simulink model "Simulink_Assem"  (R2023a)
settings: Solver=VariableStepAuto  StartTime=0.0  StopTime=10.0  RelTol=1e-3
libraries: dspsigops x1
settings Model: Creator=assem  LastModifiedBy=assem

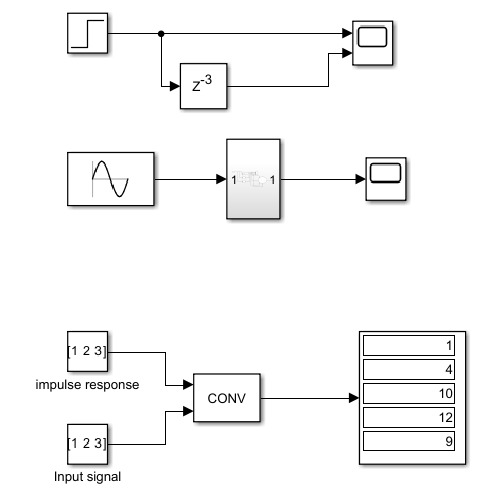
[thumbnail: Simulink's stored preview of the top-level diagram]
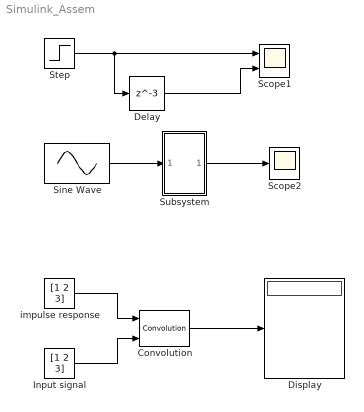
== system Simulink_Assem ==
  Convolution : dspsigops/Convolution  domain=Time  roundingMode=Floor  overflowMode=off  outputDataTypeStr=Inherit: Same as accumulator  outputMin=[]  outputMax=[]  outputLastDataTypeStr=Inherit: Same as accumulator
  Delay : Delay  DelayLength=3
  Display : Display
  Input signal : Constant  Value=[1 2 3]
  Scope1 : Scope  NumInputPorts=2
  Scope2 : Scope
  Sine Wave : Sin  SampleTime=0
  Step : Step  SampleTime=1
  Subsystem : Subsystem
  impulse response : Constant  Value=[1 2 3]
  wires:
  Step/1 -> Delay/1, Scope1/1
  impulse response/1 -> Convolution/1
  Input signal/1 -> Convolution/2
  Convolution/1 -> Display/1
  Delay/1 -> Scope1/2
  Sine Wave/1 -> Subsystem/1(In1)
  Subsystem/1(Out1) -> Scope2/1

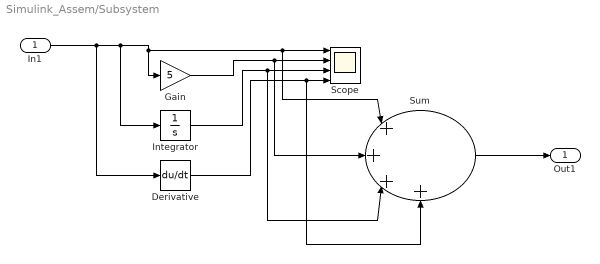
== system Simulink_Assem/Subsystem ==
  In1 : Inport
  Derivative : Derivative
  Gain : Gain  Gain=5
  Integrator : Integrator
  Scope : Scope  NumInputPorts=4
  Sum : Sum  Inputs=|++++
  Out1 : Outport
  wires:
  Sum/1 -> Out1/1
  In1/1 -> Derivative/1, Integrator/1, Gain/1, Scope/1, Sum/1
  Integrator/1 -> Sum/3, Scope/3
  Derivative/1 -> Sum/4, Scope/4
  Gain/1 -> Sum/2, Scope/2
